simulink model "navigator_barycenter"  (R2013b)
settings: Solver=FixedStepDiscrete  StartTime=0.0  StopTime=inf  FixedStep=0.2  RelTol=1e-3
undefined symbols (not defined in the file): Earth, WGS84
libraries: aerolibtransform2 x3, simulink_extras x2
settings Model: Creator=Matteo  LastModifiedBy=Gianluca Rossetti
settings OptimizationCC: OptimizeModelRefInitCode=on  LifeSpan=Inf
settings HardwareCC: ProdBitPerInt=16  ProdBitPerPointer=8  ProdIntDivRoundTo=Zero  ProdEndianess=LittleEndian  ProdWordSize=8  ProdHWDeviceType=Atmel->AVR
settings RTWCC: SystemTargetFile=ert.tlc  GenCodeOnly=on  TemplateMakefile=ert_default_tmf  Description=Embedded Coder  ProcessScript=ert_make_rtw_hook  BuildConfiguration=Faster Runs  TargetLang=C++  CheckMdlBeforeBuild=Warning
settings CodeAppCC: IgnoreCustomStorageClasses=off
settings ERTTargetCC: CodeReplacementLibrary=ANSI_C  GenerateSampleERTMain=on  ERTCustomFileTemplate=example_file_process.tlc

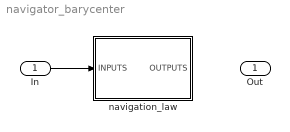
== system navigator_barycenter ==
  In : Inport  OutDataTypeStr=single  PortDimensions=21
  navigation_law : Subsystem
  Out : Outport  OutDataTypeStr=single  PortDimensions=15
  wires:
  In/1 -> navigation_law/1(INPUTS)
  ? -> Out/1

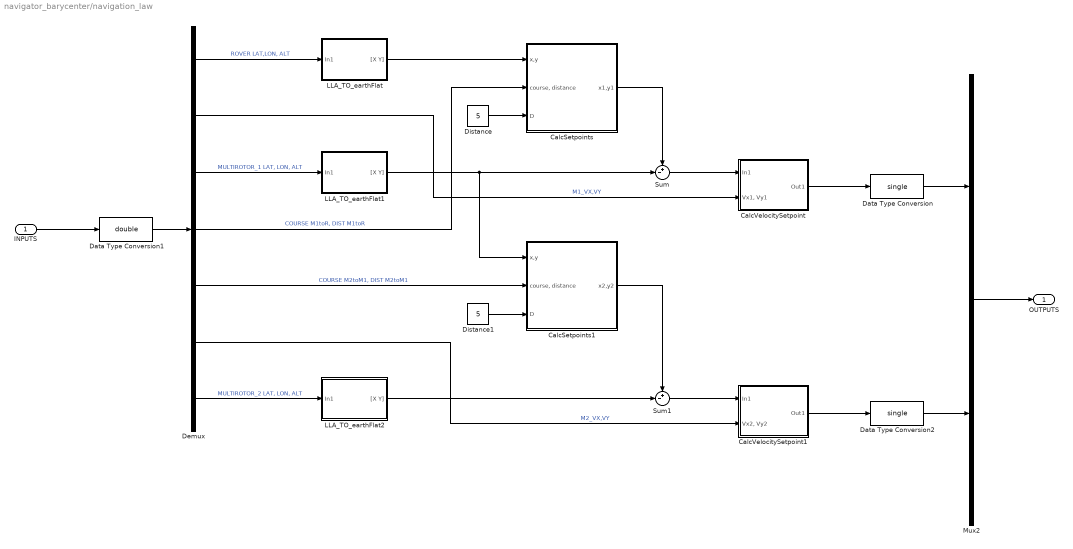
== system navigator_barycenter/navigation_law ==
  INPUTS : Inport
  CalcSetpoints : Subsystem
  CalcSetpoints1 : Subsystem
  CalcVelocitySetpoint : Subsystem
  CalcVelocitySetpoint1 : Subsystem
  Data Type Conversion : DataTypeConversion  OutDataTypeStr=single
  Data Type Conversion1 : DataTypeConversion  OutDataTypeStr=double
  Data Type Conversion2 : DataTypeConversion  OutDataTypeStr=single
  Demux : Demux  Outputs=[3 2 3 2 2 2 3]
  Distance : Constant  Value=5
  Distance1 : Constant  Value=5
  LLA_TO_earthFlat : Subsystem
  LLA_TO_earthFlat1 : Subsystem
  LLA_TO_earthFlat2 : Subsystem
  Mux2 : Mux  Inputs=[2 2]
  Sum : Sum  Inputs=+-|
  Sum1 : Sum  Inputs=+-|
  OUTPUTS : Outport
  wires:
  INPUTS/1 -> Data Type Conversion1/1
  Data Type Conversion1/1 -> Demux/1
  Demux/1 -> LLA_TO_earthFlat/1(In1)  "ROVER LAT,LON, ALT"
  Demux/2 -> CalcVelocitySetpoint/2("Vx1, Vy1")  "M1_VX,VY"
  Demux/3 -> LLA_TO_earthFlat1/1(In1)  "MULTIROTOR_1 LAT, LON, ALT"
  Demux/4 -> CalcSetpoints/2("course, distance")  "COURSE M1toR, DIST M1toR"
  Demux/7 -> LLA_TO_earthFlat2/1(In1)  "MULTIROTOR_2 LAT, LON, ALT"
  Demux/5 -> CalcSetpoints1/2("course, distance")  "COURSE M2toM1, DIST M2toM1"
  LLA_TO_earthFlat/1("[X Y]") -> CalcSetpoints/1(x,y)
  Distance/1 -> CalcSetpoints/3(D)
  LLA_TO_earthFlat1/1("[X Y]") -> CalcSetpoints1/1(x,y), Sum/2
  CalcSetpoints/1(x1,y1) -> Sum/1
  Distance1/1 -> CalcSetpoints1/3(D)
  LLA_TO_earthFlat2/1("[X Y]") -> Sum1/2
  CalcSetpoints1/1(x2,y2) -> Sum1/1
  Sum/1 -> CalcVelocitySetpoint/1(In1)
  Sum1/1 -> CalcVelocitySetpoint1/1(In1)
  Data Type Conversion/1 -> Mux2/1
  Mux2/1 -> OUTPUTS/1
  Data Type Conversion2/1 -> Mux2/2
  CalcVelocitySetpoint/1(Out1) -> Data Type Conversion/1
  CalcVelocitySetpoint1/1(Out1) -> Data Type Conversion2/1
  Demux/6 -> CalcVelocitySetpoint1/2("Vx2, Vy2")  "M2_VX,VY"

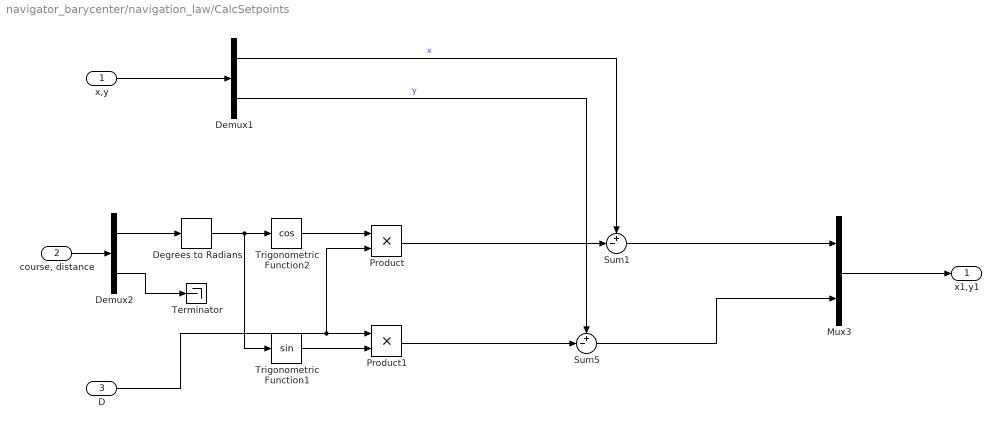
== system navigator_barycenter/navigation_law/CalcSetpoints ==
  x,y : Inport
  "course, distance" : Inport  Port=2
  D : Inport  Port=3
  Degrees to Radians : simulink_extras/Transformations/Degrees to Radians
  Demux1 : Demux  Outputs=[1 1]
  Demux2 : Demux  Outputs=[1 1]
  Mux3 : Mux  Inputs=[1 1]
  Product : Product
  Product1 : Product
  Sum1 : Sum  Inputs=+-|
  Sum5 : Sum  Inputs=+-|
  Terminator : Terminator
  Trigonometric Function1 : Trigonometry
  Trigonometric Function2 : Trigonometry  Operator=cos
  x1,y1 : Outport
  wires:
  Mux3/1 -> x1,y1/1
  Product1/1 -> Sum5/2
  "course, distance"/1 -> Demux2/1
  Demux1/2 -> Sum5/1  "y"
  Product/1 -> Sum1/2
  D/1 -> Product/2, Product1/1
  x,y/1 -> Demux1/1
  Degrees to Radians/1 -> Trigonometric Function1/1, Trigonometric Function2/1
  Trigonometric Function2/1 -> Product/1
  Trigonometric Function1/1 -> Product1/2
  Demux1/1 -> Sum1/1  "x"
  Sum1/1 -> Mux3/1
  Sum5/1 -> Mux3/2
  Demux2/1 -> Degrees to Radians/1
  Demux2/2 -> Terminator/1

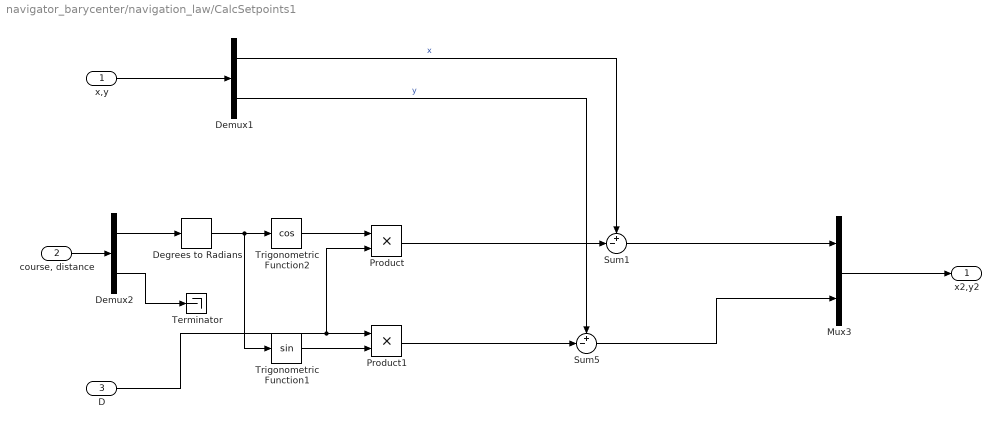
== system navigator_barycenter/navigation_law/CalcSetpoints1 ==
  x,y : Inport
  "course, distance" : Inport  Port=2
  D : Inport  Port=3
  Degrees to Radians : simulink_extras/Transformations/Degrees to Radians
  Demux1 : Demux  Outputs=[1 1]
  Demux2 : Demux  Outputs=[1 1]
  Mux3 : Mux  Inputs=[1 1]
  Product : Product
  Product1 : Product
  Sum1 : Sum  Inputs=+-|
  Sum5 : Sum  Inputs=+-|
  Terminator : Terminator
  Trigonometric Function1 : Trigonometry
  Trigonometric Function2 : Trigonometry  Operator=cos
  x2,y2 : Outport
  wires:
  Demux2/2 -> Terminator/1
  Demux2/1 -> Degrees to Radians/1
  Sum5/1 -> Mux3/2
  Sum1/1 -> Mux3/1
  Demux1/1 -> Sum1/1  "x"
  Trigonometric Function1/1 -> Product1/2
  Trigonometric Function2/1 -> Product/1
  Degrees to Radians/1 -> Trigonometric Function2/1, Trigonometric Function1/1
  x,y/1 -> Demux1/1
  D/1 -> Product1/1, Product/2
  Product/1 -> Sum1/2
  Demux1/2 -> Sum5/1  "y"
  "course, distance"/1 -> Demux2/1
  Product1/1 -> Sum5/2
  Mux3/1 -> x2,y2/1

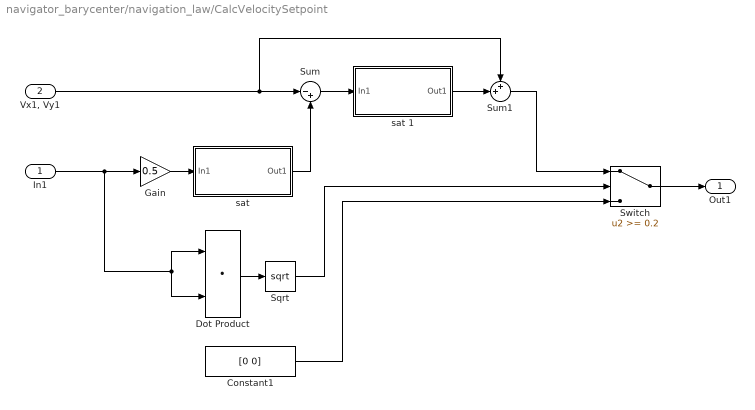
== system navigator_barycenter/navigation_law/CalcVelocitySetpoint ==
  In1 : Inport
  "Vx1, Vy1" : Inport  Port=2
  Constant1 : Constant  Value=[0 0]
  Dot Product : DotProduct  InputSameDT=on  OutDataTypeStr=Inherit: Inherit via internal rule
  Gain : Gain  Gain=0.5
  Sqrt : Sqrt  SaturateOnIntegerOverflow=on
  Sum : Sum  Inputs=|-+
  Sum1 : Sum  Inputs=++|
  Switch : Switch  Threshold=0.2
  "sat " : Subsystem  mask{k_sat=5}
      mask prompts: k_sat "Saturatore"
  sat 1 : Subsystem  mask{k_sat=5}
      mask prompts: k_sat "Saturatore"
  Out1 : Outport
  wires:
  Gain/1 -> "sat "/1(In1)
  In1/1 -> Dot Product/1, Dot Product/2, Gain/1
  Dot Product/1 -> Sqrt/1
  Sqrt/1 -> Switch/2
  "sat "/1(Out1) -> Sum/2
  Constant1/1 -> Switch/3
  Switch/1 -> Out1/1
  "Vx1, Vy1"/1 -> Sum/1, Sum1/1
  Sum/1 -> sat 1/1(In1)
  sat 1/1(Out1) -> Sum1/2
  Sum1/1 -> Switch/1

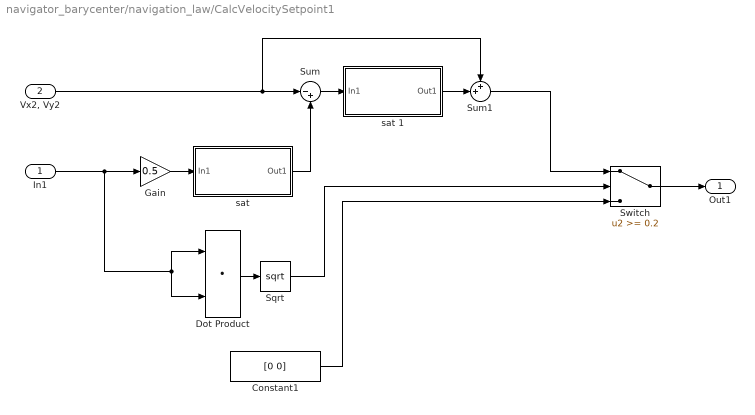
== system navigator_barycenter/navigation_law/CalcVelocitySetpoint1 ==
  In1 : Inport
  "Vx2, Vy2" : Inport  Port=2
  Constant1 : Constant  Value=[0 0]
  Dot Product : DotProduct  InputSameDT=on  OutDataTypeStr=Inherit: Inherit via internal rule
  Gain : Gain  Gain=0.5
  Sqrt : Sqrt  SaturateOnIntegerOverflow=on
  Sum : Sum  Inputs=|-+
  Sum1 : Sum  Inputs=++|
  Switch : Switch  Threshold=0.2
  "sat " : Subsystem  mask{k_sat=5}
      mask prompts: k_sat "Saturatore"
  sat 1 : Subsystem  mask{k_sat=5}
      mask prompts: k_sat "Saturatore"
  Out1 : Outport
  wires:
  Sum1/1 -> Switch/1
  sat 1/1(Out1) -> Sum1/2
  Sum/1 -> sat 1/1(In1)
  "Vx2, Vy2"/1 -> Sum1/1, Sum/1
  Switch/1 -> Out1/1
  Constant1/1 -> Switch/3
  "sat "/1(Out1) -> Sum/2
  Sqrt/1 -> Switch/2
  Dot Product/1 -> Sqrt/1
  In1/1 -> Gain/1, Dot Product/2, Dot Product/1
  Gain/1 -> "sat "/1(In1)

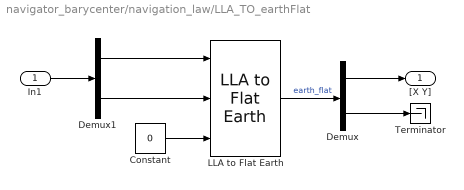
== system navigator_barycenter/navigation_law/LLA_TO_earthFlat ==
  In1 : Inport
  Constant : Constant  Value=0  OutDataTypeStr=single
  Demux : Demux  Outputs=[2 1]
  Demux1 : Demux  Outputs=[2 1]
  LLA to Flat Earth : aerolibtransform2/LLA to Flat Earth  units=Metric (MKS)  ptype=Earth (WGS84)  F=1/298.257223563  R=6378137  LL0="[44.201892800000003  12.062565800000000]"  psi=0
  Terminator : Terminator
  "[X Y]" : Outport
  wires:
  Constant/1 -> LLA to Flat Earth/3
  Demux1/1 -> LLA to Flat Earth/1
  LLA to Flat Earth/1 -> Demux/1  "earth_flat"
  Demux1/2 -> LLA to Flat Earth/2
  In1/1 -> Demux1/1
  Demux/1 -> "[X Y]"/1
  Demux/2 -> Terminator/1

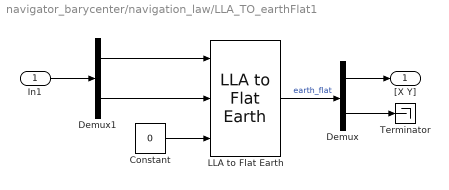
== system navigator_barycenter/navigation_law/LLA_TO_earthFlat1 ==
  In1 : Inport
  Constant : Constant  Value=0  OutDataTypeStr=single
  Demux : Demux  Outputs=[2 1]
  Demux1 : Demux  Outputs=[2 1]
  LLA to Flat Earth : aerolibtransform2/LLA to Flat Earth  units=Metric (MKS)  ptype=Earth (WGS84)  F=1/298.257223563  R=6378137  LL0="[44.201892800000003  12.062565800000000]"  psi=0
  Terminator : Terminator
  "[X Y]" : Outport
  wires:
  In1/1 -> Demux1/1
  Demux1/2 -> LLA to Flat Earth/2
  LLA to Flat Earth/1 -> Demux/1  "earth_flat"
  Demux1/1 -> LLA to Flat Earth/1
  Constant/1 -> LLA to Flat Earth/3
  Demux/1 -> "[X Y]"/1
  Demux/2 -> Terminator/1

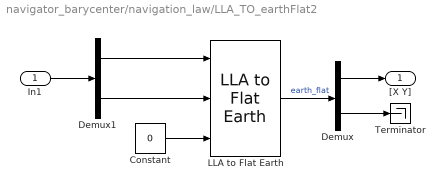
== system navigator_barycenter/navigation_law/LLA_TO_earthFlat2 ==
  In1 : Inport
  Constant : Constant  Value=0  OutDataTypeStr=single
  Demux : Demux  Outputs=[2 1]
  Demux1 : Demux  Outputs=[2 1]
  LLA to Flat Earth : aerolibtransform2/LLA to Flat Earth  units=Metric (MKS)  ptype=Earth (WGS84)  F=1/298.257223563  R=6378137  LL0="[44.201892800000003  12.062565800000000]"  psi=0
  Terminator : Terminator
  "[X Y]" : Outport
  wires:
  Constant/1 -> LLA to Flat Earth/3
  Demux1/1 -> LLA to Flat Earth/1
  LLA to Flat Earth/1 -> Demux/1  "earth_flat"
  Demux1/2 -> LLA to Flat Earth/2
  In1/1 -> Demux1/1
  Demux/1 -> "[X Y]"/1
  Demux/2 -> Terminator/1

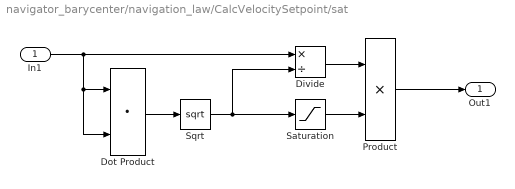
== system navigator_barycenter/navigation_law/CalcVelocitySetpoint/sat  ==
  In1 : Inport
  Divide : Product  Inputs=*/
  Dot Product : DotProduct  InputSameDT=on  OutDataTypeStr=Inherit: Inherit via internal rule
  Product : Product
  Saturation : Saturate  UpperLimit=k_sat  LowerLimit=0
  Sqrt : Sqrt  SaturateOnIntegerOverflow=on
  Out1 : Outport
  wires:
  Divide/1 -> Product/1
  Product/1 -> Out1/1
  Sqrt/1 -> Divide/2, Saturation/1
  In1/1 -> Divide/1, Dot Product/1, Dot Product/2
  Dot Product/1 -> Sqrt/1
  Saturation/1 -> Product/2

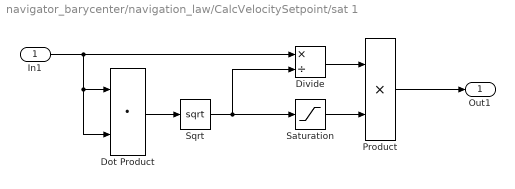
== system navigator_barycenter/navigation_law/CalcVelocitySetpoint/sat 1 ==
  In1 : Inport
  Divide : Product  Inputs=*/
  Dot Product : DotProduct  InputSameDT=on  OutDataTypeStr=Inherit: Inherit via internal rule
  Product : Product
  Saturation : Saturate  UpperLimit=k_sat  LowerLimit=0
  Sqrt : Sqrt  SaturateOnIntegerOverflow=on
  Out1 : Outport
  wires:
  Saturation/1 -> Product/2
  Dot Product/1 -> Sqrt/1
  In1/1 -> Dot Product/2, Dot Product/1, Divide/1
  Sqrt/1 -> Saturation/1, Divide/2
  Product/1 -> Out1/1
  Divide/1 -> Product/1

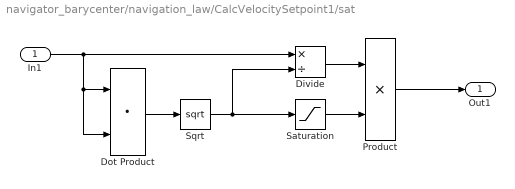
== system navigator_barycenter/navigation_law/CalcVelocitySetpoint1/sat  ==
  In1 : Inport
  Divide : Product  Inputs=*/
  Dot Product : DotProduct  InputSameDT=on  OutDataTypeStr=Inherit: Inherit via internal rule
  Product : Product
  Saturation : Saturate  UpperLimit=k_sat  LowerLimit=0
  Sqrt : Sqrt  SaturateOnIntegerOverflow=on
  Out1 : Outport
  wires:
  Saturation/1 -> Product/2
  Dot Product/1 -> Sqrt/1
  In1/1 -> Dot Product/2, Dot Product/1, Divide/1
  Sqrt/1 -> Saturation/1, Divide/2
  Product/1 -> Out1/1
  Divide/1 -> Product/1

== system navigator_barycenter/navigation_law/CalcVelocitySetpoint1/sat 1 ==
  In1 : Inport
  Divide : Product  Inputs=*/
  Dot Product : DotProduct  InputSameDT=on  OutDataTypeStr=Inherit: Inherit via internal rule
  Product : Product
  Saturation : Saturate  UpperLimit=k_sat  LowerLimit=0
  Sqrt : Sqrt  SaturateOnIntegerOverflow=on
  Out1 : Outport
  wires:
  Divide/1 -> Product/1
  Product/1 -> Out1/1
  Sqrt/1 -> Divide/2, Saturation/1
  In1/1 -> Divide/1, Dot Product/1, Dot Product/2
  Dot Product/1 -> Sqrt/1
  Saturation/1 -> Product/2
